simulink model "sim_tutorial"  (Simulink 3.00)
settings: Solver=ode23tb  StartTime=0.0  StopTime=10  RelTol=1e-3  AbsTol=1e-5
undefined symbols (not defined in the file or in its folder): a, bu, c, du, Rot
libraries: simulink3 x3

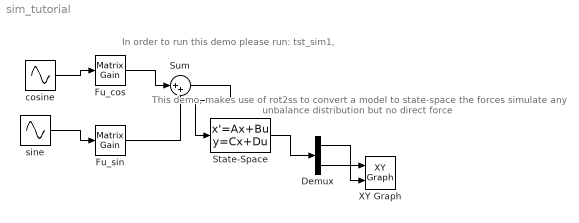
== system sim_tutorial ==
  note: In order to run this demo
      | please run:  tst_sim1,
  note: This demo, makes use of
      | rot2ss to convert a model to state-space
      | the forces simulate any unbalance distribution
      | but no direct force
  Demux : Demux  Outputs=2
  Fu_cos : simulink3/Math/Matrix Gain  K=Rot.Fu_cos
  Fu_sin : simulink3/Math/Matrix Gain  K=Rot.Fu_sin
  State-Space : StateSpace  A=a  B=bu  C=c  D=du  X0=0
  Sum : Sum  Inputs=|++  SaturateOnIntegerOverflow=on
  XY Graph : simulink3/Sinks/XY Graph  xmin=-2e-6  xmax=2e-6  ymin=-2e-6  ymax=2e-6  st=-1
  cosine : Sin  Amplitude=1  Frequency=Rot.W  Phase=pi/2  SampleTime=0
  sine : Sin  Amplitude=1  Frequency=Rot.W  Phase=0  SampleTime=0
  wires:
  cosine/1 -> Fu_cos/1
  sine/1 -> Fu_sin/1
  Sum/1 -> State-Space/1
  Fu_cos/1 -> Sum/1
  Fu_sin/1 -> Sum/2
  Demux/1 -> XY Graph/1
  Demux/2 -> XY Graph/2
  State-Space/1 -> Demux/1
